simulink model "simple_PP"  (Simulink 8.5)
settings: Solver=VariableStepDiscrete  StartTime=0.0  StopTime=10.0  RelTol=1e-3
settings Model: Creator=arnaud  LastModifiedBy=shizue  CovSFcnEnable=off
settings DataIOCC: SaveFormat=Structure
settings DebuggingCC: SolverPrmCheckMsg=warning  FcnCallInpInsideContextMsg=EnableAllAsWarning

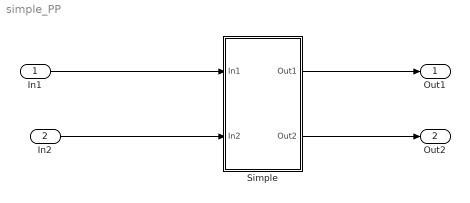
== system simple_PP ==
  In1 : Inport
  In2 : Inport  Port=2
  "Simple " : Subsystem  TreatAsAtomicUnit=on
  Out1 : Outport
  Out2 : Outport  Port=2
  wires:
  In1/1 -> "Simple "/1(In1)
  In2/1 -> "Simple "/2(In2)
  "Simple "/1(Out1) -> Out1/1
  "Simple "/2(Out2) -> Out2/1

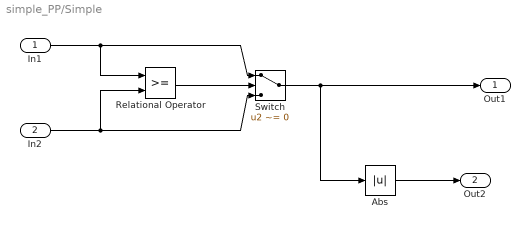
== system simple_PP/Simple  ==
  In1 : Inport
  In2 : Inport  Port=2
  Abs : Abs
  Relational Operator : RelationalOperator  OutDataTypeStr=boolean
  Switch : Switch  Criteria=u2 ~= 0
  Out1 : Outport
  Out2 : Outport  Port=2
  wires:
  Switch/1 -> Out1/1, Abs/1
  Abs/1 -> Out2/1
  In1/1 -> Relational Operator/1, Switch/1
  Relational Operator/1 -> Switch/2
  In2/1 -> Relational Operator/2, Switch/3
